simulink model "PID_controller_project"  (R2017a)
settings: Solver=VariableStepAuto  StartTime=0.0  StopTime=20  RelTol=1e-3
values from neighbouring files (symbols this model uses):
  Kd = input('Enter with a new differential gain (Kd): ')    [PID_controller_project.m]
  Ki = input('Enter with a new integral gain (Ki): ')    [PID_controller_project.m]
  Kp = 0.6*Km    [PID_controller_project.m]
undefined symbols (not defined in the file or in its folder): den, num
settings Model: Creator=Marcos  LastModifiedBy=Marcos

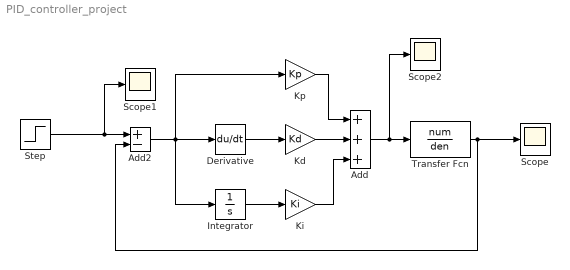
== system PID_controller_project ==
  Add : Sum  Inputs=+++
  Add2 : Sum  Inputs=+-
  Derivative : Derivative
  Integrator : Integrator
  "Kd " : Gain  Gain=Kd
  Ki : Gain  Gain=Ki
  Kp : Gain  Gain=Kp
  Scope : Scope
  Scope1 : Scope
  Scope2 : Scope
  Step : Step  After=30  SampleTime=2
  Transfer Fcn : TransferFcn  Numerator=num  Denominator=den
  wires:
  Integrator/1 -> Ki/1
  Derivative/1 -> "Kd "/1
  "Kd "/1 -> Add/2
  Add2/1 -> Integrator/1, Kp/1, Derivative/1
  Step/1 -> Scope1/1, Add2/1
  Kp/1 -> Add/1
  Ki/1 -> Add/3
  Add/1 -> Scope2/1, Transfer Fcn/1
  Transfer Fcn/1 -> Scope/1, Add2/2
